simulink model "ex2"  (R2015b)
settings: Solver=VariableStepAuto  StartTime=0.0  StopTime=10  RelTol=1e-3
settings Model: Creator=ovi  LastModifiedBy=ovi

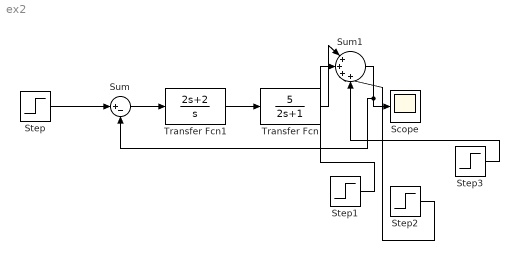
== system ex2 ==
  Scope : Scope
  Step : Step  SampleTime=0
  Step1 : Step  Time=2  After=0.2  SampleTime=0
  Step2 : Step  Time=4  After=0.3  SampleTime=0
  Step3 : Step  Time=6  After=0.4  SampleTime=0
  Sum : Sum  Inputs=|+-
  Sum1 : Sum  Inputs=|++++
  Transfer Fcn : TransferFcn  Numerator=[5]  Denominator=[2 1]
  Transfer Fcn1 : TransferFcn  Numerator=[2 2]  Denominator=[1 0]
  wires:
  Sum/1 -> Transfer Fcn1/1
  Step/1 -> Sum/1
  Transfer Fcn1/1 -> Transfer Fcn/1
  Step1/1 -> Sum1/2
  Transfer Fcn/1 -> Sum1/1
  Sum1/1 -> Sum/2, Scope/1
  Step2/1 -> Sum1/3
  Step3/1 -> Sum1/4
